simulink model "Sim"  (R2017a)
settings: Solver=VariableStepAuto  StartTime=0.0  StopTime=3e-3  RelTol=1e-3
values from neighbouring files (symbols this model uses):
  dz = 1    [initial.m]
  gl = 0.3    [initial.m]
  ri = 10    [initial.m]
  ro = 10    [initial.m]
libraries: fl_lib x14, nesl_utility x4
settings Model: Creator=faezeh  LastModifiedBy=faezeh

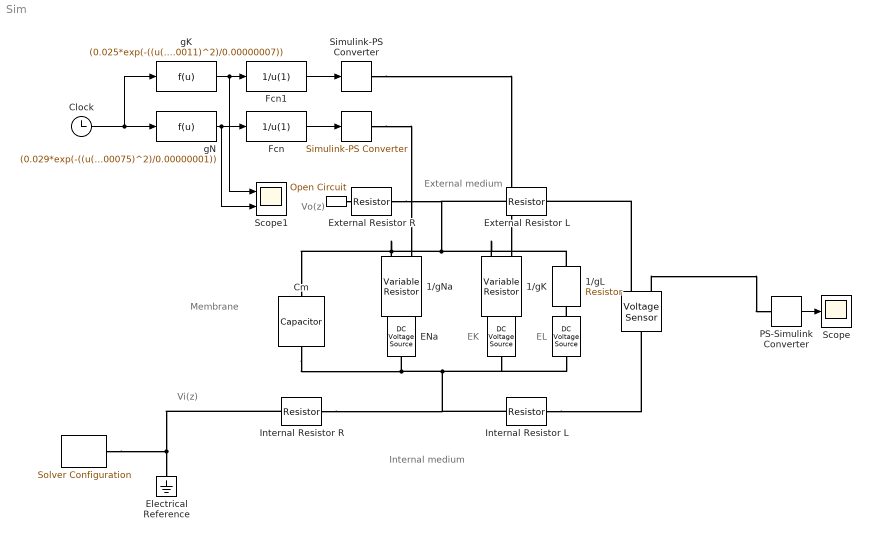
== system Sim ==
  note: External medium
  note: Internal medium
  note: EL
  note: EK
  note: Vi(z)
  note: Vo(z)
  note: Membrane
  " " : fl_lib/Electrical/Electrical Sources/DC Voltage Source  v0=El mV
  "  " : fl_lib/Electrical/Electrical Elements/Open Circuit  v_specify=on  v_priority=None  v=Vr mV  v_nominal_specify=off  v_nominal_unit=V  v_nominal_value=1
      settings: SourceProductName=Simscape  SourceProductBaseCode=SS
  "    " : nesl_utility/Simulink-PS Converter  PhysicalDomain=network_engine_domain  SubClassName=ps_input  LeftPortType=input  RightPortType=output  PseudoPeriodic=off  Frequencies=[]  NoiseDistribution=none  NoiseParameters=[]  Unit=1  AffineConversion=off  FilteringAndDerivatives=provide  SimscapeFilterOrder=1  InputFilterTimeConstant=0.001  UdotUserProvided=0
  "     " : fl_lib/Electrical/Electrical Sources/DC Voltage Source  v0=Ek mV
  "      " : nesl_utility/Solver Configuration  PhysicalDomain=network_engine_domain  SubClassName=solver  LeftPortType=input  RightPortType=generic  Accelerate=off  Tones=[]  Harmonics=[]  SimulateNoise=off  Profile=off  UseLocalSampling=off  EnableSwitchedLinearOptims=on  FrequencyDomain=off  UseCCode=off  RelTol=0.001  AbsTol=1e-06  MinStep=1e-09  ToWorkspace=off  RevertToSquareIcSolve=off  NumHomotopyIterations=100  PhasorMode=off  PhasorModeNumHarmonics=1  OverrideAbsTol=off  DoDC=off  ResidualTolerance=1e-09  UseLocalSolver=off  LocalSolverChoice=NE_BACKWARD_EULER_ADVANCER  LocalSolverSampleTime=0.001  DoFixedCost=off  MaxNonlinIter=3  MaxModeIter=2  LinearAlgebra=Sparse  DelaysMemoryBudget=1024  AutomaticFiltering=on  FilteringTimeConstant=0.001
  "       " : fl_lib/Electrical/Electrical Sensors/Voltage Sensor
  " External Resistor L" : fl_lib/Electrical/Electrical Elements/Resistor  R=ro*(dz/2) Ohm  i_specify=off  i_priority=None  i=0 A  i_nominal_specify=off  i_nominal_unit=A  i_nominal_value=1  v_specify=off  v_priority=None  v=0 V  v_nominal_specify=off  v_nominal_unit=V  v_nominal_value=1
  " External Resistor R" : fl_lib/Electrical/Electrical Elements/Resistor  R=ro*(dz/2) Ohm  i_specify=off  i_priority=None  i=0 A  i_nominal_specify=off  i_nominal_unit=A  i_nominal_value=1  v_specify=off  v_priority=None  v=0 V  v_nominal_specify=off  v_nominal_unit=V  v_nominal_value=1
  " Internal Resistor L" : fl_lib/Electrical/Electrical Elements/Resistor  R=ri*(dz/2) Ohm  i_specify=off  i_priority=None  i=0 A  i_nominal_specify=off  i_nominal_unit=A  i_nominal_value=1  v_specify=off  v_priority=None  v=0 V  v_nominal_specify=off  v_nominal_unit=V  v_nominal_value=1
  " Internal Resistor R" : fl_lib/Electrical/Electrical Elements/Resistor  R=ri*(dz/2) Ohm  i_specify=off  i_priority=None  i=0 A  i_nominal_specify=off  i_nominal_unit=A  i_nominal_value=1  v_specify=off  v_priority=None  v=0 V  v_nominal_specify=off  v_nominal_unit=V  v_nominal_value=1
  1/gK : fl_lib/Electrical/Electrical Elements/Variable Resistor  Rmin=0 Ohm  i_specify=off  i_priority=None  i=0 A  i_nominal_specify=off  i_nominal_unit=A  i_nominal_value=1  v_specify=off  v_priority=None  v=0 V  v_nominal_specify=off  v_nominal_unit=V  v_nominal_value=1
  1/gL : fl_lib/Electrical/Electrical Elements/Resistor  R=1/gl Ohm  i_specify=off  i_priority=None  i=0 A  i_nominal_specify=off  i_nominal_unit=A  i_nominal_value=1  v_specify=off  v_priority=None  v=0 V  v_nominal_specify=off  v_nominal_unit=V  v_nominal_value=1
  1/gNa : fl_lib/Electrical/Electrical Elements/Variable Resistor  Rmin=0 Ohm  i_specify=off  i_priority=None  i=0 A  i_nominal_specify=off  i_nominal_unit=A  i_nominal_value=1  v_specify=off  v_priority=None  v=0 V  v_nominal_specify=off  v_nominal_unit=V  v_nominal_value=1
  Clock : Clock
  Cm : fl_lib/Electrical/Electrical Elements/Capacitor  c=Cm uF  r=1e-6 Ohm  g=0 1/Ohm  i_specify=off  i_priority=None  i=0 A  i_nominal_specify=off  i_nominal_unit=A  i_nominal_value=1  v_specify=off  v_priority=None  v=0 V  v_nominal_specify=off  v_nominal_unit=V  v_nominal_value=1  vc_specify=off  vc_priority=High  vc=0 V  vc_nominal_specify=off  vc_nominal_unit=V  vc_nominal_value=1
  ENa : fl_lib/Electrical/Electrical Sources/DC Voltage Source  v0=Ena mV
  Electrical Reference : fl_lib/Electrical/Electrical Elements/Electrical Reference
  Fcn : Fcn  Expr=1/u(1)
  Fcn1 : Fcn  Expr=1/u(1)
  PS-Simulink Converter : nesl_utility/PS-Simulink Converter  PhysicalDomain=network_engine_domain  SubClassName=ps_output  LeftPortType=input  RightPortType=output  PseudoPeriodic=off  Frequencies=[]  Unit=1  AffineConversion=off
  Scope : Scope
  Scope1 : Scope  NumInputPorts=2
  Simulink-PS Converter : nesl_utility/Simulink-PS Converter  PhysicalDomain=network_engine_domain  SubClassName=ps_input  LeftPortType=input  RightPortType=output  PseudoPeriodic=off  Frequencies=[]  NoiseDistribution=none  NoiseParameters=[]  Unit=1  AffineConversion=off  FilteringAndDerivatives=provide  SimscapeFilterOrder=1  InputFilterTimeConstant=0.001  UdotUserProvided=0
  gK : Fcn  Expr=(0.025*exp(-((u(1)-0.0011)^2)/0.00000007))
  gN : Fcn  Expr=(0.029*exp(-((u(1)-0.00075)^2)/0.00000001))
  wires:
  PS-Simulink Converter/1 -> Scope/1
  Clock/1 -> gN/1, gK/1
  gN/1 -> Scope1/2, Fcn/1
  Fcn/1 -> "    "/1
  gK/1 -> Scope1/1, Fcn1/1
  Fcn1/1 -> Simulink-PS Converter/1
  connections:
  1/gL/LConn1 -- 1/gK/LConn2 -- " External Resistor L"/LConn1 -- " External Resistor R"/RConn1 -- 1/gNa/LConn2 -- Cm/LConn1
  Cm/RConn1 -- " Internal Resistor R"/LConn1 -- " Internal Resistor L"/RConn1 -- " "/RConn1 -- "     "/RConn1 -- ENa/LConn1
  " "/LConn1 -- 1/gL/RConn1
  "       "/RConn1 -- PS-Simulink Converter/LConn1
  "      "/RConn1 -- " Internal Resistor R"/RConn1 -- Electrical Reference/LConn1
  "     "/LConn1 -- 1/gK/RConn1
  ENa/RConn1 -- 1/gNa/RConn1
  "       "/RConn2 -- " External Resistor L"/RConn1
  Simulink-PS Converter/RConn1 -- 1/gK/LConn1
  "    "/RConn1 -- 1/gNa/LConn1
  " Internal Resistor L"/LConn1 -- "       "/LConn1
  "  "/LConn1 -- " External Resistor R"/LConn1
